simulink subsystem "ideal_coldend"  (R2022b)
settings: Solver=VariableStepAuto  StartTime=0.0  StopTime=10.0  RelTol=1e-3
undefined symbols (not defined in the file or in its folder): ambient
libraries: fl_lib x5, nesl_utility x1
settings Model: Creator=wilde  LastModifiedBy=wilde

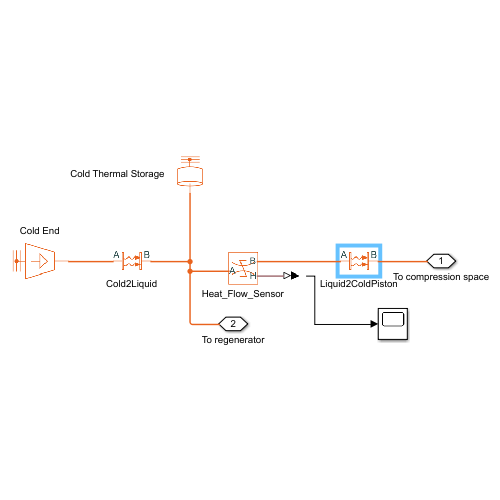
[thumbnail: Simulink's stored preview of the top-level diagram]
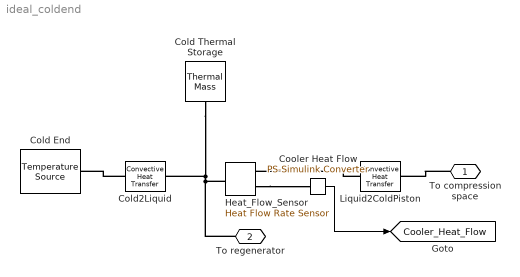
== system ideal_coldend ==
  Cold End : fl_lib/Thermal/Thermal Sources/Temperature Source  temperature=ambient.temperature K
  Cold Thermal Storage : fl_lib/Thermal/Thermal Elements/Thermal Mass  mass=ambient.fins.m kg  sp_heat=ambient.fins.cp J/(K*kg)  num_ports=foundation.enum.numPorts2.one  T_specify=on  T_priority=High  T=ambient.fins.T.init K  T_nominal_specify=off  T_nominal_unit=K  T_nominal_value=1  Q_specify=off  Q_priority=None  Q=0 W  Q_nominal_specify=off  Q_nominal_unit=W  Q_nominal_value=1
  Cold2Liquid : fl_lib/Thermal/Thermal Elements/Convective Heat Transfer  thermal_type=foundation.enum.constant_variable.constant  area=a.ambient.fins.area m^2  heat_tr_coeff=a.ambient.fins.h W/(K*m^2)  min_heat_tr_coeff=1e-3 W/(K*m^2)  T_specify=off  T_priority=None  T=0 K  T_nominal_specify=off  T_nominal_unit=K  T_nominal_value=1  Q_specify=off  Q_priority=None  Q=0 W  Q_nominal_specify=off  Q_nominal_unit=W  Q_nominal_value=1
  Cooler Heat Flow : nesl_utility/PS-Simulink Converter  PhysicalDomain=network_engine_domain  SubClassName=ps_output  LeftPortType=input  RightPortType=output  PseudoPeriodic=off  Frequencies=[]  VectorFormat=inherit  Unit=inherit  AffineConversion=off
  Heat_Flow_Sensor : fl_lib/Thermal/Thermal Sensors/Heat Flow Rate Sensor
  Liquid2ColdPiston : fl_lib/Thermal/Thermal Elements/Convective Heat Transfer  thermal_type=foundation.enum.constant_variable.constant  area=a.ambient.fins.area m^2  heat_tr_coeff=a.ambient.fins.h W/(K*m^2)  min_heat_tr_coeff=1e-3 W/(K*m^2)  T_specify=off  T_priority=None  T=0 K  T_nominal_specify=off  T_nominal_unit=K  T_nominal_value=1  Q_specify=off  Q_priority=None  Q=0 W  Q_nominal_specify=off  Q_nominal_unit=W  Q_nominal_value=1
  To compression space : PMIOPort  Side=Left
  To regenerator : PMIOPort  Port=2  Side=Left
  tag scope: Cooler_Heat_Flow=global
  wires:
  Cooler Heat Flow/1 -> [Cooler_Heat_Flow]
  connections:
  Heat_Flow_Sensor/LConn1 -- To regenerator/RConn1 -- Cold2Liquid/RConn1 -- Cold Thermal Storage/LConn1
  To compression space/RConn1 -- Liquid2ColdPiston/RConn1
  Heat_Flow_Sensor/RConn1 -- Cooler Heat Flow/LConn1
  Liquid2ColdPiston/LConn1 -- Heat_Flow_Sensor/RConn2
  Cold2Liquid/LConn1 -- Cold End/LConn1
